simulink model "r2_1f_2x_4a_4k_r366"  (R2012b)
(part 4 of 95)

  xeng0/3(valid) -> vacc_tvg0/4(valid_in), snap_xeng0/2(we)
  [xeng_tvg_sel] -> xeng_tvg0/1(tvg_sel)
  [vacc_tvg_sel] -> vacc_tvg0/1(tvg_sel)
  Delay151/1(q) -> Delay83/1(d)
  Delay20/1(q) -> xeng_tvg0/2(sync)
  Delay21/1(q) -> xeng_tvg0/3(data_in)
  Delay22/1(q) -> xeng_tvg0/4(valid_in)
  Delay26/1(q) -> Delay151/1(d)
  gbe_rx_err_cnt0/1(sim_out) -> Terminator7/1
  Delay2/1(q) -> gbe_rx_err_cnt0/1(out_reg)
  Subsystem/2(rx_err_cnt) -> Delay2/1(d)
  Slice2/1 -> Delay117/1(d)
  Delay117/1(q) -> [loopback_mux_rst]
  Delay118/1(q) -> negedge_delay1/1(in)
  Slice8/1 -> Delay122/1(d)
  Delay122/1(q) -> [gbe_out_rst]
  16b_32b/1(Out1) -> snap_xeng0/1(din), vacc_tvg0/3(data_in)
  last_missing_ant0/1(sim_out) -> Terminator11/1
  Delay130/1(q) -> last_missing_ant0/1(out_reg)
  miss_cnt0/3(last_missed_ant) -> Convert2/1
  Slice14/1 -> Delay100/1(d)
  Delay100/1(q) -> [gbe_out_enable]
  spead_unpack0/8(hdr3_0x4102) -> pre_process0/7(hdr3)
  spead_unpack0/5(pkt_bad) -> Delay82/1(d), pre_process0/4(spead_err)
  Delay12/1(q) -> Subsystem4/8(overrun)
  [gbe_up0] -> Delay87/1(d)
  [gbe_rx0] -> Delay86/1(d)
  [gbe_rxvld0] -> delay46/1
  [gbe_rxdata0] -> delay45/1
  [gbe_rxeof0] -> delay47/1
  Delay87/1(q) -> Subsystem4/1(led_up)
  Delay86/1(q) -> Subsystem4/2(led_rx)
  delay45/1 -> spead_unpack0/1(pkt_data)
  delay46/1 -> spead_unpack0/2(pkt_valid)
  delay47/1 -> spead_unpack0/3(pkt_eof)
  vacc_tvg0/1(sync_out) -> vacc0/5(sync_in)
  vacc_tvg0/2(data_out) -> vacc0/6(data_in)
  vacc_tvg0/3(valid_out) -> vacc0/7(we)
  [acc_len] -> vacc0/4(acc_len)
  xeng0/4(mcnt_out) -> delay5/1
  vacc_cnt0/1(sim_out) -> Terminator10/1
  vacc_monitor/2(spec_cnt) -> vacc_cnt0/1(out_reg)
  vacc_err_cnt0/1(sim_out) -> Terminator1/1
  vacc_monitor/1(error_cnt) -> vacc_err_cnt0/1(out_reg)
  vacc0/1(new_acc) -> [new_acc0]
  [cnt_rst] -> vacc_monitor/1(cnt_rst)
  vacc0/7(timestamp) -> delay7/1
  [gbe_up0] -> Subsystem3/5(link_up)
  [gbe_tx0] -> Subsystem3/6(led_tx)
  [gbe_txd0] -> Subsystem3/1(data_in)
  [gbe_txvld0] -> Subsystem3/2(valid_in)
  [gbe_txip] -> Subsystem3/3(ip_in)
  [gbe_txeof0] -> Subsystem3/4(eof_in)
  [gbe_rxvld0] -> Delay25/1(d)
  [gbe_rxeof0] -> Delay18/1(d)
  Delay25/1(q) -> Subsystem/2(valid)
  Delay18/1(q) -> Subsystem/3(eof)
  [gbe_rx_bad0] -> Delay6/1(d)
  [gbe_rx_over0] -> Delay7/1(d)
  [gbe_rxip0] -> Delay53/1(d)
  [gbe_rxvld0] -> Delay59/1(d)
  [gbe_rxdata0] -> Delay70/1(d)
  [gbe_rxeof0] -> Delay29/1(d)
  Delay70/1(q) -> Subsystem4/3(data_in)
  Delay59/1(q) -> Subsystem4/4(valid_in)
  Delay53/1(q) -> Subsystem4/5(ip_in)
  Delay29/1(q) -> Subsystem4/6(eof_in)
  Constant1/1 -> Delay103/1(d)
  Delay80/1(q) -> Subsystem5/2(we)
  Delay81/1(q) -> Subsystem5/3(eof)
  Delay82/1(q) -> Subsystem5/4(flag)
  [gbe_tx_over0] -> gbe_err/4(overflow)
  [gbe_txeof0] -> gbe_err/3(eof)
  [gbe_txvld0] -> gbe_err/2(valid)
  Delay6/1(q) -> Subsystem/4(rx_bad_frame)
  Delay7/1(q) -> Subsystem/5(rx_overflow)
  [gbe_rx_bad0] -> Delay8/1(d)
  [gbe_rx_over0] -> Delay12/1(d)
  [gbe_tx_full0] -> Subsystem3/7(tx_full)
  [gbe_tx_over0] -> Subsystem3/8(tx_over)
  Delay56/1(q) -> xeng0/1(sync_in)
  Delay73/1(q) -> xeng0/2(ant)
  Delay74/1(q) -> xeng0/3(window_valid)
  Delay83/1(q) -> xeng0/4(mcnt_in)
  [gbe_out_rst] -> delay8/1
  [gbe_txd0] -> delay9/1
  [gbe_txvld0] -> delay10/1
  [gbe_txip] -> delay11/1
  [gbe_txport] -> delay12/1
  [gbe_txeof0] -> delay13/1
  gbe0/1 -> [gbe_up0]
  gbe0/2 -> [gbe_rx0]
  gbe0/3 -> [gbe_tx0]
  gbe0/4 -> [gbe_tx_full0]
  gbe0/5 -> [gbe_tx_over0]
  gbe0/12 -> [gbe_rx_over0]
  gbe0/11 -> [gbe_rx_bad0]
  gbe0/6 -> [gbe_rxdata0]
  gbe0/7 -> [gbe_rxvld0]
  gbe0/8 -> [gbe_rxip0]
  gbe0/9 -> [gbe_rxport0]
  gbe0/10 -> [gbe_rxeof0]
  [vacc_ld_arm] -> vacc0/2(arm)
  [vacc_ld_time] -> vacc0/3(load_time)
  [vacc_rst] -> vacc0/1(rst)
  vacc_ld_status0/1(sim_out) -> Terminator4/1
  delay5/1 -> vacc0/8(pcnt_in)
  vacc0/10(error_out) -> [vacc_err0]
  [new_acc0] -> vacc_monitor/2(new_acc)
  [vacc_err0] -> vacc_monitor/3(error)
  pkt_reord_devel2/2(data_out) -> snap_reord0/2(in_data), Delay21/1(d)
  Delay27/1(q) -> negedge_delay2/1(in)
  Delay96/1(q) -> negedge_delay3/1(in)
  Delay97/1(q) -> negedge_delay4/1(in)
  miss_cnt0/4(not_rcvd) -> [xeng_rx_err0]
  vacc0/2(data_out) -> delay4/1
  vacc0/4(valid_out) -> delay2/1
  vacc0/6(rb_done) -> delay6/1
  [vacc_ld_stat0] -> vacc_ld_status0/1(out_reg)
  vacc0/8(ld_status) -> [vacc_ld_stat0]
  [id0] -> pack_out0/6(xeng_id)
  [vacc_err0] -> snap_vacc0/4(stop)
  pack_out0/3(eof) -> Delay15/1(d)
  pack_out_err0/1(sim_out) -> Terminator6/1
  pack_out_cnt0/1(sim_out) -> Terminator5/1
  [cnt_rst] -> vacc_monitor2/1(cnt_rst)
  vacc_monitor2/1(pkt_cnt) -> pack_out_cnt0/1(out_reg)
  vacc_monitor2/2(error_cnt) -> pack_out_err0/1(out_reg)
  pack_out0/5(fetch) -> vacc0/9(re)
  delay4/1 -> snap_vacc0/1(din), pack_out0/1(data_in)
  delay2/1 -> snap_vacc0/2(we), pack_out0/2(valid_in)
  delay6/1 -> pack_out0/4(rb_done), snap_vacc0/3(trig)
  delay7/1 -> pack_out0/5(timestamp)
  pack_out0/1(data_out) -> Delay23/1(d)
  pack_out0/2(valid_out) -> Logical/2
  pack_out0/4(err) -> Delay34/1(d)
  Delay34/1(q) -> [pack_err0], vacc_monitor2/3(error)
  delay8/1 -> gbe0/1
  delay9/1 -> gbe0/2
  delay10/1 -> gbe0/3
  delay11/1 -> gbe0/4
  delay12/1 -> gbe0/5
  delay13/1 -> gbe0/6
  Constant2/1 -> gbe0/7
  Constant8/1 -> gbe0/8
  Delay46/1 -> pack_out0/3(pkt_rdy)
  Slice6/1 -> Delay44/1(d)
  Delay44/1(q) -> [flasher_en]
  negedge_delay3/1(out) -> front_panel/6(led2_red)
  negedge_delay4/1(out) -> front_panel/7(led3_red)
  [flasher_en] -> front_panel/1(flasher_en)
  [new_acc0] -> front_panel/2(sync)
  [x_sync0] -> front_panel/3(step)
  xstatus0/1(sim_out) -> Terminator24/1
  Subsystem6/1(status) -> xstatus0/1(out_reg)
  [clr_status] -> Subsystem6/1(clr)
  negedge_delay2/1(out) -> front_panel/4(led0_red)
  negedge_delay/1(out) -> front_panel/10(led6_green)
  negedge_delay1/1(out) -> front_panel/9(led5_green)
  Slice10/1 -> Delay13/1(d)
  Delay13/1(q) -> [clr_status]
  Inverter5/1 -> Subsystem6/2(gbe_down)
  [gbe_up0] -> Inverter5/1
  [vacc_err0] -> Subsystem6/10(vacc_err)
  [gbe_rx_bad0] -> Subsystem6/12(rx_bad_frame)
  [pack_err0] -> Subsystem6/15(pack_err)
  Subsystem3/1(data_out) -> snap_gbe_tx0/1(din)
  Subsystem3/2(we_out) -> snap_gbe_tx0/2(we)
  Subsystem3/3(trig_out) -> snap_gbe_tx0/3(trig)
  Subsystem4/1(data_out) -> snap_gbe_rx0/1(din)
  Subsystem4/2(we_out) -> snap_gbe_rx0/2(we)
  Subsystem4/3(trig_out) -> snap_gbe_rx0/3(trig)
  Delay16/1 -> [gbe_txvld0]
  Delay23/1(q) -> rate_ctrl0/1(din0)
  rate_ctrl0/2(valid) -> Delay16/1
  Constant22/1 -> [beng_data_id]
  rate_ctrl0/1(dout) -> Delay114/1
  Delay114/1 -> [gbe_txd0]
  err_clear_sim1/1 -> gbe_out_port/1(sim_1)
  gbe_out_port/1(in_reg) -> Delay9/1(d)
  Delay9/1(q) -> [gbe_out_txport]
  err_clear_sim5/1 -> gbe_out_ip/1(sim_1)
  gbe_out_ip/1(in_reg) -> Delay10/1(d)
  Delay10/1(q) -> [gbe_out_ip_addr]
  [gbe_out_txport] -> [gbe_txport]
  [gbe_out_ip_addr] -> [gbe_txip]
  [gbe_out_enable] -> Logical/1
  Constant24/1 -> [beng_time_id]
  Logical/1 -> rate_ctrl0/2(valid0)
  Delay15/1(q) -> vacc_monitor2/2(eof), rate_ctrl0/3(eof0)
  vacc0/5(pkt_rdy) -> rate_ctrl0/4(data_rdy0)
  spead_unpack0/1(pkt_start) -> Terminator28/1
  spead_unpack0/9(hdr4_0x4103) -> pre_process0/8(hdr4)
  pre_process0/9(dest_err) -> [rx_dest_err0]
  pre_process0/1(data_out) -> pkt_reord_devel2/1(din)
  pre_process0/2(valid) -> pkt_reord_devel2/2(valid_in)
  pre_process0/3(eof_out) -> pkt_reord_devel2/3(eof)
  pre_process0/4(timestamp) -> pkt_reord_devel2/4(time)
  pre_process0/5(feng_id) -> pkt_reord_devel2/5(ant)
  pre_process0/6(freq_out) -> pkt_reord_devel2/6(freq)
  pre_process0/8(spead_err_out) -> [spead_err0]
  pre_process0/7(adc_over) -> [adc_err0]
  pre_process0/10(fft_err) -> [fft_err0]
  pre_process0/11(feng_rx_err) -> [feng_rx_err0]
  pre_process0/12(nd_en) -> [noise_diode_en0]
  pkt_reord_devel2/7(err) -> Terminator2/1
  pre_process0/13(chksum_err) -> [feng_chk_err0]
  pre_process0/14(qdr_err) -> [feng_qdr_err0]
  [id0] -> pre_process0/9(board_id)
  err_clear_sim3/1 -> board_id/1(sim_1)
  Constant3/1 -> Delay72/1(d)
  Delay72/1(q) -> Subsystem1/1(In1)
  Subsystem1/1(Out1) -> [id0]
  Subsystem1/2(Out2) -> [id1]
  Subsystem1/3(Out3) -> [id2]
  Subsystem1/4(Out4) -> [id3]
  [id0] -> pkt_reord_devel2/8(board_id)
  pkt_reord_devel2/3(valid_out) -> snap_reord0/10(we), snap_reord0/3(in_valid), miss_cnt0/3(valid), Logical6/2, Delay22/1(d)
  pkt_reord_devel2/5(freq_out) -> Convert12/1
  Slice12/1 -> snap_reord0/7(in_feng_err)
  Slice16/1 -> snap_reord0/9(in_nd_on)
  Slice15/1 -> snap_reord0/8(in_adc_over)
  pkt_reord_devel2/6(flag_out) -> Slice11/1, Slice12/1, Slice15/1, Slice16/1
  Slice11/1 -> Logical6/1, snap_reord0/6(in_xeng_err), miss_cnt0/4(not rcvd)
  Logical6/1 -> snap_reord0/12(stop)
  miss_cnt1/2(missing_cnt) -> Convert4/1
  [cnt_rst] -> miss_cnt1/1(rst)
  miss_cnt1/1(spectr_cnt) -> Convert3/1
  pkt_reord_devel1/4(time_out) -> Slice21/1, Delay30/1(d)
  pkt_reord_devel1/1(sync_out) -> snap_reord1/11(trig), snap_reord1/1(in_sync), miss_cnt1/2(sync), Delay5/1(d)
  xeng_tvg1/1(sync_out) -> Delay32/1(d)
  xeng_tvg1/2(data_out) -> Delay36/1(d)
  xeng_tvg1/3(valid_out) -> Delay37/1(d)
  xeng1/1(sync_out) -> vacc_tvg1/2(sync_in)
  xeng1/2(acc) -> 16b_32b1/1(In1)
  xeng1/3(valid) -> vacc_tvg1/4(valid_in)
  [xeng_tvg_sel] -> xeng_tvg1/1(tvg_sel)
  [vacc_tvg_sel] -> vacc_tvg1/1(tvg_sel)
  Delay4/1(q) -> Delay38/1(d)
  Delay5/1(q) -> xeng_tvg1/2(sync)
  Delay11/1(q) -> xeng_tvg1/3(data_in)
  Delay14/1(q) -> xeng_tvg1/4(valid_in)
  Delay30/1(q) -> Delay4/1(d)
  16b_32b1/1(Out1) -> vacc_tvg1/3(data_in)
  miss_cnt1/3(last_missed_ant) -> Convert5/1
  vacc_tvg1/1(sync_out) -> vacc1/5(sync_in)
  vacc_tvg1/2(data_out) -> vacc1/6(data_in)
  vacc_tvg1/3(valid_out) -> vacc1/7(we)
  [acc_len] -> vacc1/4(acc_len)
  xeng1/4(mcnt_out) -> delay16/1
  vacc_monitor1/2(spec_cnt) -> vacc_cnt1/1(out_reg)
  vacc_monitor1/1(error_cnt) -> vacc_err_cnt1/1(out_reg)
  vacc1/1(new_acc) -> vacc_monitor1/2(new_acc), [new_acc1]
  [cnt_rst] -> vacc_monitor1/1(cnt_rst)
  vacc1/7(timestamp) -> delay18/1
  Delay32/1(q) -> xeng1/1(sync_in)
  Delay36/1(q) -> xeng1/2(ant)
  Delay37/1(q) -> xeng1/3(window_valid)
  Delay38/1(q) -> xeng1/4(mcnt_in)
  [vacc_ld_arm] -> vacc1/2(arm)
  [vacc_ld_time] -> vacc1/3(load_time)
  [vacc_rst] -> vacc1/1(rst)
  delay16/1 -> vacc1/8(pcnt_in)
  pkt_reord_devel1/2(data_out) -> snap_reord1/2(in_data), Delay11/1(d)
  miss_cnt1/4(not_rcvd) -> [xeng_rx_err1]
  vacc1/2(data_out) -> delay3/1
  vacc1/4(valid_out) -> delay1/1
  vacc1/6(rb_done) -> delay17/1
  vacc1/5(pkt_rdy) -> rate_ctrl1/4(data_rdy0)
  vacc1/8(ld_status) -> vacc_ld_status1/1(out_reg)
  [id1] -> pack_out1/6(xeng_id)
  vacc1/10(error_out) -> snap_vacc1/4(stop), vacc_monitor1/3(error), [vacc_err1]
  pack_out1/3(eof) -> Delay3/1(d)
  pack_out_err1/1(sim_out) -> Terminator31/1
  pack_out_cnt1/1(sim_out) -> Terminator29/1
  [cnt_rst] -> vacc_monitor3/1(cnt_rst)
  vacc_monitor3/1(pkt_cnt) -> pack_out_cnt1/1(out_reg)
  vacc_monitor3/2(error_cnt) -> pack_out_err1/1(out_reg)
  pack_out1/5(fetch) -> vacc1/9(re)
  delay3/1 -> pack_out1/1(data_in), snap_vacc1/1(din)
  delay1/1 -> pack_out1/2(valid_in), snap_vacc1/2(we)
  delay17/1 -> pack_out1/4(rb_done), snap_vacc1/3(trig)
  delay18/1 -> pack_out1/5(timestamp)
  pack_out1/1(data_out) -> Delay28/1(d)
  pack_out1/2(valid_out) -> Logical7/2
  Delay28/1(q) -> rate_ctrl1/1(din0)
  Logical7/1 -> rate_ctrl1/2(valid0)
  pack_out1/4(err) -> Delay31/1(d)
  Delay3/1(q) -> vacc_monitor3/2(eof), rate_ctrl1/3(eof0)
  Delay31/1(q) -> [pack_err1], vacc_monitor3/3(error)
  Delay42/1 -> pack_out1/3(pkt_rdy)
  [gbe_out_enable] -> Logical7/1
  pkt_reord_devel1/7(err) -> Terminator20/1
  [id1] -> pkt_reord_devel1/8(board_id)
  [flags1] -> pkt_reord_devel1/7(flag)
  pkt_reord_devel1/3(valid_out) -> snap_reord1/10(we), snap_reord1/3(in_valid), miss_cnt1/3(valid), Logical8/2, Delay14/1(d)
  pkt_reord_devel1/5(freq_out) -> Convert13/1
  Slice18/1 -> snap_reord1/7(in_feng_err)
  Slice20/1 -> snap_reord1/9(in_nd_on)
  Slice19/1 -> snap_reord1/8(in_adc_over)
  pkt_reord_devel1/6(flag_out) -> Slice20/1, Slice19/1, Slice18/1, Slice17/1
  Slice17/1 -> snap_reord1/6(in_xeng_err), miss_cnt1/4(not rcvd), Logical8/1
  Logical8/1 -> snap_reord1/12(stop)
  Constant12/1 -> vacc_time_msw/1(sim_1)
  Constant6/1 -> vacc_time_lsw/1(sim_1)
  vacc_time_msw/1(in_reg) -> Slice4/1, Slice13/1
  Slice13/1 -> Concat12/1
  vacc_time_lsw/1(in_reg) -> Concat12/2
  Slice4/1 -> [vacc_ld_arm]
  Concat12/1 -> [vacc_ld_time]
  rate_ctrl0/3(eof) -> Delay45/1
  rate_ctrl0/4(pkt_send0) -> Delay46/1
  Delay45/1 -> [gbe_txeof0]
  Delay40/1 -> [gbe_txvld1]
  rate_ctrl1/2(valid) -> Delay40/1
  rate_ctrl1/1(dout) -> Delay39/1
  Delay39/1 -> [gbe_txd1]
  rate_ctrl1/3(eof) -> Delay41/1
  rate_ctrl1/4(pkt_send0) -> Delay42/1
  Delay41/1 -> [gbe_txeof1]
  Subsystem8/1(rx_cnt) -> Delay68/1(d)
  [cnt_rst] -> Subsystem8/1(rst)
  spead_unpack1/3(valid64) -> Delay85/1(d), pre_process1/2(valid_in)
  spead_unpack1/6(hdr1_0x1600) -> pre_process1/5(hdr1)
  spead_unpack1/2(data64) -> pre_process1/1(data_in)
  spead_unpack1/4(eof64) -> Delay90/1(d), pre_process1/3(eof_in)
  spead_unpack1/7(hdr2_0x4101) -> pre_process1/6(hdr2)
  Subsystem8/2(err_cnt) -> Delay69/1(d)
  rx_cnt1/1(sim_out) -> Terminator32/1
  rx_err_cnt1/1(sim_out) -> Terminator33/1
  spead_unpack1/8(hdr3_0x4102) -> pre_process1/7(hdr3)
  spead_unpack1/5(pkt_bad) -> Delay91/1(d), pre_process1/4(spead_err)
  gbe1/6 -> Delay84/1(d)
  Delay84/1(q) -> spead_unpack1/1(pkt_data)
  Delay77/1(q) -> spead_unpack1/2(pkt_valid)
  Delay57/1(q) -> spead_unpack1/3(pkt_eof)
  Delay85/1(q) -> Subsystem8/2(we)
  Delay90/1(q) -> Subsystem8/3(eof)
  Delay91/1(q) -> Subsystem8/4(flag)
  spead_unpack1/1(pkt_start) -> Terminator34/1
  spead_unpack1/9(hdr4_0x4103) -> pre_process1/8(hdr4)
  pre_process1/9(dest_err) -> [rx_dest_err1]
  pre_process1/1(data_out) -> pkt_reord_devel1/1(din)
  pre_process1/2(valid) -> pkt_reord_devel1/2(valid_in)
  pre_process1/3(eof_out) -> pkt_reord_devel1/3(eof)
  pre_process1/4(timestamp) -> pkt_reord_devel1/4(time)
  pre_process1/5(feng_id) -> pkt_reord_devel1/5(ant)
  pre_process1/6(freq_out) -> pkt_reord_devel1/6(freq)
  pre_process1/8(spead_err_out) -> [spead_err1]
  pre_process1/7(adc_over) -> [adc_err1]
  pre_process1/10(fft_err) -> [fft_err1]
  pre_process1/11(feng_rx_err) -> [feng_rx_err1]
  pre_process1/12(nd_en) -> [noise_diode_en1]
  pre_process1/13(chksum_err) -> [feng_chk_err1]
  pre_process1/14(qdr_err) -> [feng_qdr_err1]
  [id1] -> pre_process1/9(board_id)
  [gbe_out_rst] -> delay21/1
  [gbe_txd1] -> delay22/1
  [gbe_txip] -> delay15/1
  [gbe_txport] -> delay19/1
  delay21/1 -> gbe1/1
  delay22/1 -> gbe1/2
  delay14/1 -> gbe1/3
  delay15/1 -> gbe1/4
  delay19/1 -> gbe1/5
  delay20/1 -> gbe1/6
  Constant9/1 -> gbe1/7
  Constant13/1 -> gbe1/8
  gbe_err1/1(tx_cnt) -> Delay98/1(d)
  Subsystem9/1(rx_cnt) -> Delay101/1(d)
  [cnt_rst] -> gbe_err1/1(rst)
  [cnt_rst] -> Subsystem9/1(rst)
  gbe_err1/2(err_cnt) -> Delay99/1(d)
  gbe_rx_cnt1/1(sim_out) -> Terminator37/1
  Delay98/1(q) -> gbe_tx_cnt1/1(out_reg)
  Delay99/1(q) -> gbe_tx_err_cnt1/1(out_reg)
  Delay101/1(q) -> gbe_rx_cnt1/1(out_reg)
  gbe_rx_err_cnt1/1(sim_out) -> Terminator38/1
  Delay93/1(q) -> gbe_rx_err_cnt1/1(out_reg)
  Subsystem9/2(rx_err_cnt) -> Delay93/1(d)
  gbe1/7 -> Delay94/1(d), Delay77/1(d)
  gbe1/10 -> Delay57/1(d), Delay92/1(d)
  Delay94/1(q) -> Subsystem9/2(valid)
  Delay92/1(q) -> Subsystem9/3(eof)
  gbe1/11 -> Delay95/1(d), [gbe_rx_bad1]
  gbe1/12 -> Delay102/1(d)
  gbe1/5 -> [gbe_tx_over1], gbe_err1/4(overflow)
  [gbe_txeof1] -> gbe_err1/3(eof), delay20/1
  [gbe_txvld1] -> gbe_err1/2(valid), delay14/1
  Delay95/1(q) -> Subsystem9/4(rx_bad_frame)
  Delay102/1(q) -> Subsystem9/5(rx_overflow)
  Delay103/1(q) -> Subsystem4/9(ack_in)
  miss_cnt2/2(missing_cnt) -> Convert7/1
  [cnt_rst] -> miss_cnt2/1(rst)
  miss_cnt2/1(spectr_cnt) -> Convert6/1
  pkt_reord_devel3/4(time_out) -> Slice27/1, Delay111/1(d)
  pkt_reord_devel3/1(sync_out) -> Delay133/1(d), snap_reord2/11(trig), snap_reord2/1(in_sync), miss_cnt2/2(sync)
  xeng_tvg2/1(sync_out) -> Delay113/1(d)
  xeng_tvg2/2(data_out) -> Delay119/1(d)
  xeng_tvg2/3(valid_out) -> Delay120/1(d)
  xeng2/1(sync_out) -> vacc_tvg2/2(sync_in)
  xeng2/2(acc) -> 16b_32b2/1(In1)
  xeng2/3(valid) -> vacc_tvg2/4(valid_in)
  [xeng_tvg_sel] -> xeng_tvg2/1(tvg_sel)
  [vacc_tvg_sel] -> vacc_tvg2/1(tvg_sel)
  Delay124/1(q) -> Delay121/1(d)
  Delay133/1(q) -> xeng_tvg2/2(sync)
  Delay107/1(q) -> xeng_tvg2/3(data_in)
  Delay108/1(q) -> xeng_tvg2/4(valid_in)
  Delay111/1(q) -> Delay124/1(d)
  16b_32b2/1(Out1) -> vacc_tvg2/3(data_in)
  miss_cnt2/3(last_missed_ant) -> Convert8/1
  vacc_tvg2/1(sync_out) -> vacc2/5(sync_in)
  vacc_tvg2/2(data_out) -> vacc2/6(data_in)
  vacc_tvg2/3(valid_out) -> vacc2/7(we)
  [acc_len] -> vacc2/4(acc_len)
  xeng2/4(mcnt_out) -> delay26/1
  vacc_cnt2/1(sim_out) -> Terminator55/1
  vacc_monitor4/2(spec_cnt) -> vacc_cnt2/1(out_reg)
  vacc_err_cnt2/1(sim_out) -> Terminator46/1
  vacc_monitor4/1(error_cnt) -> vacc_err_cnt2/1(out_reg)
  vacc2/1(new_acc) -> [new_acc2], vacc_monitor4/2(new_acc)
  [cnt_rst] -> vacc_monitor4/1(cnt_rst)
  vacc2/7(timestamp) -> delay28/1
  Delay113/1(q) -> xeng2/1(sync_in)
  Delay119/1(q) -> xeng2/2(ant)
  Delay120/1(q) -> xeng2/3(window_valid)
  Delay121/1(q) -> xeng2/4(mcnt_in)
  [vacc_ld_arm] -> vacc2/2(arm)
  [vacc_ld_time] -> vacc2/3(load_time)
  [vacc_rst] -> vacc2/1(rst)
  vacc_ld_status2/1(sim_out) -> Terminator43/1
  delay26/1 -> vacc2/8(pcnt_in)
  pkt_reord_devel3/2(data_out) -> snap_reord2/2(in_data), Delay107/1(d)
  miss_cnt2/4(not_rcvd) -> [xeng_rx_err2]
  vacc2/2(data_out) -> delay33/1
  vacc2/4(valid_out) -> delay23/1
  vacc2/6(rb_done) -> delay27/1
  vacc2/5(pkt_rdy) -> rate_ctrl2/4(data_rdy0)
  vacc2/8(ld_status) -> vacc_ld_status2/1(out_reg)
  [id2] -> pack_out2/6(xeng_id)
  vacc2/10(error_out) -> [vacc_err2], vacc_monitor4/3(error), snap_vacc2/4(stop)
  pack_out2/3(eof) -> Delay110/1(d)
  pack_out_err2/1(sim_out) -> Terminator47/1
  pack_out_cnt2/1(sim_out) -> Terminator45/1
  [cnt_rst] -> vacc_monitor5/1(cnt_rst)
  vacc_monitor5/1(pkt_cnt) -> pack_out_cnt2/1(out_reg)
  vacc_monitor5/2(error_cnt) -> pack_out_err2/1(out_reg)
  pack_out2/5(fetch) -> vacc2/9(re)
  delay33/1 -> snap_vacc2/1(din), pack_out2/1(data_in)
  delay23/1 -> snap_vacc2/2(we), pack_out2/2(valid_in)
  delay27/1 -> snap_vacc2/3(trig), pack_out2/4(rb_done)
  delay28/1 -> pack_out2/5(timestamp)
  pack_out2/1(data_out) -> Delay109/1(d)
  pack_out2/2(valid_out) -> Logical12/2
  Delay109/1(q) -> rate_ctrl2/1(din0)
  Logical12/1 -> rate_ctrl2/2(valid0)
  pack_out2/4(err) -> Delay112/1(d)
  Delay110/1(q) -> rate_ctrl2/3(eof0), vacc_monitor5/2(eof)
  Delay112/1(q) -> [pack_err2], vacc_monitor5/3(error)
  Delay127/1 -> pack_out2/3(pkt_rdy)
  [gbe_out_enable] -> Logical12/1
  pkt_reord_devel3/7(err) -> Terminator40/1
  [id2] -> pkt_reord_devel3/8(board_id)
  [flags2] -> pkt_reord_devel3/7(flag)
  pkt_reord_devel3/3(valid_out) -> Delay108/1(d), Logical13/2, snap_reord2/10(we), miss_cnt2/3(valid), snap_reord2/3(in_valid)
  pkt_reord_devel3/5(freq_out) -> Convert14/1
  Slice24/1 -> snap_reord2/7(in_feng_err)
  Slice26/1 -> snap_reord2/9(in_nd_on)
  Slice25/1 -> snap_reord2/8(in_adc_over)
  pkt_reord_devel3/6(flag_out) -> Slice26/1, Slice25/1, Slice23/1, Slice24/1
  Slice23/1 -> Logical13/1, snap_reord2/6(in_xeng_err), miss_cnt2/4(not rcvd)
  Logical13/1 -> snap_reord2/12(stop)
  Delay125/1 -> [gbe_txvld2]
  rate_ctrl2/2(valid) -> Delay125/1
  rate_ctrl2/1(dout) -> Delay123/1
  Delay123/1 -> [gbe_txd2]
  rate_ctrl2/3(eof) -> Delay126/1
  rate_ctrl2/4(pkt_send0) -> Delay127/1
  Delay126/1 -> [gbe_txeof2]
  Subsystem11/1(rx_cnt) -> Delay149/1(d)
  [cnt_rst] -> Subsystem11/1(rst)
  spead_unpack2/3(valid64) -> pre_process2/2(valid_in), Delay155/1(d)
  spead_unpack2/6(hdr1_0x1600) -> pre_process2/5(hdr1)
  spead_unpack2/2(data64) -> pre_process2/1(data_in)
  spead_unpack2/4(eof64) -> pre_process2/3(eof_in), Delay156/1(d)
  spead_unpack2/7(hdr2_0x4101) -> pre_process2/6(hdr2)
  Subsystem11/2(err_cnt) -> Delay150/1(d)
  rx_cnt2/1(sim_out) -> Terminator48/1
  rx_err_cnt2/1(sim_out) -> Terminator49/1
  Delay149/1(q) -> rx_cnt2/1(out_reg)
  Delay150/1(q) -> rx_err_cnt2/1(out_reg)
  spead_unpack2/8(hdr3_0x4102) -> pre_process2/7(hdr3)
  spead_unpack2/5(pkt_bad) -> pre_process2/4(spead_err), Delay157/1(d)
  gbe2/6 -> Delay154/1(d)
  Delay154/1(q) -> spead_unpack2/1(pkt_data)
  Delay153/1(q) -> spead_unpack2/2(pkt_valid)
  Delay139/1(q) -> spead_unpack2/3(pkt_eof)
  Delay155/1(q) -> Subsystem11/2(we)
  Delay156/1(q) -> Subsystem11/3(eof)
  Delay157/1(q) -> Subsystem11/4(flag)
  spead_unpack2/1(pkt_start) -> Terminator50/1
  spead_unpack2/9(hdr4_0x4103) -> pre_process2/8(hdr4)
  pre_process2/9(dest_err) -> [rx_dest_err2]
  pre_process2/1(data_out) -> pkt_reord_devel3/1(din)
  pre_process2/2(valid) -> pkt_reord_devel3/2(valid_in)
  pre_process2/3(eof_out) -> pkt_reord_devel3/3(eof)
  pre_process2/4(timestamp) -> pkt_reord_devel3/4(time)
  pre_process2/5(feng_id) -> pkt_reord_devel3/5(ant)
  pre_process2/6(freq_out) -> pkt_reord_devel3/6(freq)
  pre_process2/8(spead_err_out) -> [spead_err2]
  pre_process2/7(adc_over) -> [adc_err2]
  pre_process2/10(fft_err) -> [fft_err2]
  pre_process2/11(feng_rx_err) -> [feng_rx_err2]
  pre_process2/12(nd_en) -> [noise_diode_en2]
  pre_process2/13(chksum_err) -> [feng_chk_err2]
  pre_process2/14(qdr_err) -> [feng_qdr_err2]
  [id2] -> pre_process2/9(board_id)
  [gbe_out_rst] -> delay31/1
  [gbe_txd2] -> delay32/1
  [gbe_txip] -> delay25/1
  [gbe_txport] -> delay29/1
  delay31/1 -> gbe2/1
  delay32/1 -> gbe2/2
  delay24/1 -> gbe2/3
  delay25/1 -> gbe2/4
  delay29/1 -> gbe2/5
  delay30/1 -> gbe2/6
  Constant18/1 -> gbe2/7
  Constant14/1 -> gbe2/8
  gbe_err2/1(tx_cnt) -> Delay162/1(d)
  Subsystem12/1(rx_cnt) -> Delay105/1(d)
  [cnt_rst] -> gbe_err2/1(rst)
  [cnt_rst] -> Subsystem12/1(rst)
  gbe_err2/2(err_cnt) -> Delay163/1(d)
  gbe_tx_cnt2/1(sim_out) -> Terminator51/1
  gbe_tx_err_cnt2/1(sim_out) -> Terminator52/1
  gbe_rx_cnt2/1(sim_out) -> Terminator53/1
  Delay162/1(q) -> gbe_tx_cnt2/1(out_reg)
  Delay163/1(q) -> gbe_tx_err_cnt2/1(out_reg)
  Delay105/1(q) -> gbe_rx_cnt2/1(out_reg)
  gbe_rx_err_cnt2/1(sim_out) -> Terminator54/1
  Delay159/1(q) -> gbe_rx_err_cnt2/1(out_reg)
  Subsystem12/2(rx_err_cnt) -> Delay159/1(d)
  gbe2/7 -> Delay153/1(d), Delay160/1(d)
  gbe2/10 -> Delay158/1(d), Delay139/1(d)
  Delay160/1(q) -> Subsystem12/2(valid)
  Delay158/1(q) -> Subsystem12/3(eof)
  gbe2/11 -> [gbe_rx_bad2], Delay161/1(d)
  gbe2/12 -> Delay106/1(d)
  gbe2/5 -> [gbe_tx_over2], gbe_err2/4(overflow)
  [gbe_txeof2] -> delay30/1, gbe_err2/3(eof)
  [gbe_txvld2] -> delay24/1, gbe_err2/2(valid)
  Delay161/1(q) -> Subsystem12/4(rx_bad_frame)
  Delay106/1(q) -> Subsystem12/5(rx_overflow)
  miss_cnt3/2(missing_cnt) -> Convert10/1
  [cnt_rst] -> miss_cnt3/1(rst)
  miss_cnt3/1(spectr_cnt) -> Convert9/1
  pkt_reord_devel4/4(time_out) -> Slice36/1, Delay171/1(d)
  pkt_reord_devel4/1(sync_out) -> Delay188/1(d), snap_reord3/11(trig), snap_reord3/1(in_sync), miss_cnt3/2(sync)
  xeng_tvg3/1(sync_out) -> Delay173/1(d)
  xeng_tvg3/2(data_out) -> Delay176/1(d)
  xeng_tvg3/3(valid_out) -> Delay177/1(d)
  xeng3/1(sync_out) -> vacc_tvg3/2(sync_in)
  xeng3/2(acc) -> 16b_32b3/1(In1)
  xeng3/3(valid) -> vacc_tvg3/4(valid_in)
  [xeng_tvg_sel] -> xeng_tvg3/1(tvg_sel)
  [vacc_tvg_sel] -> vacc_tvg3/1(tvg_sel)
  Delay180/1(q) -> Delay178/1(d)
  Delay188/1(q) -> xeng_tvg3/2(sync)
  Delay167/1(q) -> xeng_tvg3/3(data_in)
  Delay168/1(q) -> xeng_tvg3/4(valid_in)
  Delay171/1(q) -> Delay180/1(d)
  16b_32b3/1(Out1) -> vacc_tvg3/3(data_in)
  miss_cnt3/3(last_missed_ant) -> Convert11/1
  vacc_tvg3/1(sync_out) -> vacc3/5(sync_in)
  vacc_tvg3/2(data_out) -> vacc3/6(data_in)
  vacc_tvg3/3(valid_out) -> vacc3/7(we)
  [acc_len] -> vacc3/4(acc_len)
  xeng3/4(mcnt_out) -> delay37/1
  vacc_monitor6/2(spec_cnt) -> vacc_cnt3/1(out_reg)
  vacc_monitor6/1(error_cnt) -> vacc_err_cnt3/1(out_reg)
  vacc3/1(new_acc) -> vacc_monitor6/2(new_acc), [new_acc3]
  [cnt_rst] -> vacc_monitor6/1(cnt_rst)
  vacc3/7(timestamp) -> delay39/1
  Delay173/1(q) -> xeng3/1(sync_in)
  Delay176/1(q) -> xeng3/2(ant)
  Delay177/1(q) -> xeng3/3(window_valid)
  Delay178/1(q) -> xeng3/4(mcnt_in)
  [vacc_ld_arm] -> vacc3/2(arm)
  [vacc_ld_time] -> vacc3/3(load_time)
  [vacc_rst] -> vacc3/1(rst)
  delay37/1 -> vacc3/8(pcnt_in)
  pkt_reord_devel4/2(data_out) -> snap_reord3/2(in_data), Delay167/1(d)
  miss_cnt3/4(not_rcvd) -> [xeng_rx_err3]
  vacc3/2(data_out) -> delay44/1
  vacc3/4(valid_out) -> delay34/1
  vacc3/6(rb_done) -> delay38/1
  vacc3/5(pkt_rdy) -> rate_ctrl3/4(data_rdy0)
  vacc3/8(ld_status) -> vacc_ld_status3/1(out_reg)
  [id3] -> pack_out3/6(xeng_id)
  vacc3/10(error_out) -> snap_vacc3/4(stop), vacc_monitor6/3(error), [vacc_err3]
  pack_out3/3(eof) -> Delay170/1(d)
  pack_out_err3/1(sim_out) -> Terminator64/1
  pack_out_cnt3/1(sim_out) -> Terminator62/1
  [cnt_rst] -> vacc_monitor7/1(cnt_rst)
  vacc_monitor7/1(pkt_cnt) -> pack_out_cnt3/1(out_reg)
  vacc_monitor7/2(error_cnt) -> pack_out_err3/1(out_reg)
  pack_out3/5(fetch) -> vacc3/9(re)
  delay44/1 -> pack_out3/1(data_in), snap_vacc3/1(din)
  delay34/1 -> pack_out3/2(valid_in), snap_vacc3/2(we)
  delay38/1 -> pack_out3/4(rb_done), snap_vacc3/3(trig)
  delay39/1 -> pack_out3/5(timestamp)
  pack_out3/1(data_out) -> Delay169/1(d)
  pack_out3/2(valid_out) -> Logical16/2
  Delay169/1(q) -> rate_ctrl3/1(din0)
  Logical16/1 -> rate_ctrl3/2(valid0)
  pack_out3/4(err) -> Delay172/1(d)
  Delay170/1(q) -> vacc_monitor7/2(eof), rate_ctrl3/3(eof0)
  Delay172/1(q) -> [pack_err3], vacc_monitor7/3(error)
  Delay183/1 -> pack_out3/3(pkt_rdy)
  [gbe_out_enable] -> Logical16/1
  pkt_reord_devel4/7(err) -> Terminator57/1
  [id3] -> pkt_reord_devel4/8(board_id)
  [flags3] -> pkt_reord_devel4/7(flag)
  pkt_reord_devel4/3(valid_out) -> snap_reord3/10(we), snap_reord3/3(in_valid), miss_cnt3/3(valid), Logical17/2, Delay168/1(d)
  pkt_reord_devel4/5(freq_out) -> Convert15/1
  Slice33/1 -> snap_reord3/7(in_feng_err)
  Slice35/1 -> snap_reord3/9(in_nd_on)
  Slice34/1 -> snap_reord3/8(in_adc_over)
  pkt_reord_devel4/6(flag_out) -> Slice35/1, Slice34/1, Slice33/1, Slice32/1
  Slice32/1 -> snap_reord3/6(in_xeng_err), miss_cnt3/4(not rcvd), Logical17/1
  Logical17/1 -> snap_reord3/12(stop)
  Delay181/1 -> [gbe_txvld3]
  rate_ctrl3/2(valid) -> Delay181/1
  rate_ctrl3/1(dout) -> Delay179/1
  Delay179/1 -> [gbe_txd3]
  rate_ctrl3/3(eof) -> Delay182/1
  rate_ctrl3/4(pkt_send0) -> Delay183/1
  Delay182/1 -> [gbe_txeof3]
  Subsystem14/1(rx_cnt) -> Delay195/1(d)
  [cnt_rst] -> Subsystem14/1(rst)
  spead_unpack3/3(valid64) -> pre_process3/2(valid_in), Delay200/1(d)
  spead_unpack3/6(hdr1_0x1600) -> pre_process3/5(hdr1)
  spead_unpack3/2(data64) -> pre_process3/1(data_in)
  spead_unpack3/4(eof64) -> pre_process3/3(eof_in), Delay201/1(d)
  spead_unpack3/7(hdr2_0x4101) -> pre_process3/6(hdr2)
  Subsystem14/2(err_cnt) -> Delay196/1(d)
  Delay195/1(q) -> rx_cnt3/1(out_reg)
  Delay196/1(q) -> rx_err_cnt3/1(out_reg)
  spead_unpack3/8(hdr3_0x4102) -> pre_process3/7(hdr3)
  spead_unpack3/5(pkt_bad) -> pre_process3/4(spead_err), Delay202/1(d)
  gbe3/6 -> Delay199/1(d)
  Delay199/1(q) -> spead_unpack3/1(pkt_data)
  Delay198/1(q) -> spead_unpack3/2(pkt_valid)
  Delay194/1(q) -> spead_unpack3/3(pkt_eof)
  Delay200/1(q) -> Subsystem14/2(we)
  Delay201/1(q) -> Subsystem14/3(eof)
  Delay202/1(q) -> Subsystem14/4(flag)
  spead_unpack3/1(pkt_start) -> Terminator67/1
  spead_unpack3/9(hdr4_0x4103) -> pre_process3/8(hdr4)
  pre_process3/9(dest_err) -> [rx_dest_err3], snap_unpack3/9(in_dest_err), Logical1/2
  pre_process3/1(data_out) -> snap_unpack3/1(in_data), pkt_reord_devel4/1(din)
  pre_process3/2(valid) -> snap_unpack3/2(in_valid), snap_unpack3/15(we), pkt_reord_devel4/2(valid_in)
  pre_process3/3(eof_out) -> pkt_reord_devel4/3(eof), snap_unpack3/16(trig), snap_unpack3/3(in_eof)
  pre_process3/4(timestamp) -> pkt_reord_devel4/4(time), Slice29/1
  pre_process3/5(feng_id) -> pkt_reord_devel4/5(ant), Slice30/1
  pre_process3/6(freq_out) -> pkt_reord_devel4/6(freq), Slice31/1
  pre_process3/8(spead_err_out) -> snap_unpack3/8(in_spead_err), Logical1/1, [spead_err3]
  pre_process3/7(adc_over) -> snap_unpack3/7(in_adc_over), [adc_err3]
  pre_process3/11(feng_rx_err) -> snap_unpack3/11(in_feng_rx_err), [feng_rx_err3]
  pre_process3/12(nd_en) -> snap_unpack3/12(in_nd_en), [noise_diode_en3]
  pre_process3/13(chksum_err) -> snap_unpack3/13(in_chksum_err), [feng_chk_err3]
  pre_process3/14(qdr_err) -> [feng_qdr_err3], snap_unpack3/14(in_feng_qdr_err)
  [id3] -> pre_process3/9(board_id)
  [gbe_out_rst] -> delay42/1
  [gbe_txd3] -> delay43/1
  [gbe_txip] -> delay36/1
  [gbe_txport] -> delay40/1
  delay42/1 -> gbe3/1
  delay43/1 -> gbe3/2
  delay35/1 -> gbe3/3
  delay36/1 -> gbe3/4
  delay40/1 -> gbe3/5
  delay41/1 -> gbe3/6
  Constant23/1 -> gbe3/7
  Constant19/1 -> gbe3/8
  gbe_err3/1(tx_cnt) -> Delay207/1(d)
  Subsystem15/1(rx_cnt) -> Delay165/1(d)
  [cnt_rst] -> gbe_err3/1(rst)
  [cnt_rst] -> Subsystem15/1(rst)
  gbe_err3/2(err_cnt) -> Delay208/1(d)
  gbe_tx_cnt3/1(sim_out) -> Terminator68/1
  gbe_tx_err_cnt3/1(sim_out) -> Terminator69/1
  gbe_rx_cnt3/1(sim_out) -> Terminator70/1
  Delay207/1(q) -> gbe_tx_cnt3/1(out_reg)
  Delay208/1(q) -> gbe_tx_err_cnt3/1(out_reg)
  Delay165/1(q) -> gbe_rx_cnt3/1(out_reg)
  gbe_rx_err_cnt3/1(sim_out) -> Terminator71/1
  Delay204/1(q) -> gbe_rx_err_cnt3/1(out_reg)
  Subsystem15/2(rx_err_cnt) -> Delay204/1(d)
  gbe3/7 -> Delay205/1(d), Delay198/1(d)
  gbe3/10 -> Delay194/1(d), Delay203/1(d)
  Delay205/1(q) -> Subsystem15/2(valid)
  Delay203/1(q) -> Subsystem15/3(eof)
  gbe3/11 -> [gbe_rx_bad3], Delay206/1(d)
  gbe3/12 -> Delay166/1(d)
  gbe3/5 -> [gbe_tx_over3], gbe_err3/4(overflow)
  [gbe_txeof3] -> gbe_err3/3(eof), delay41/1
  [gbe_txvld3] -> gbe_err3/2(valid), delay35/1
  Delay206/1(q) -> Subsystem15/4(rx_bad_frame)
  Delay166/1(q) -> Subsystem15/5(rx_overflow)
  gbe1/1 -> [gbe_up1]
  gbe2/1 -> [gbe_up2]
  gbe3/1 -> [gbe_up3]
  [spead_err0] -> Subsystem6/11(rx_bad_pkt)
  [xeng_rx_err0] -> Subsystem6/14(xeng_bad_dat)
  [gbe_tx_over0] -> Subsystem6/13(tx_over)
  [rx_dest_err0] -> Subsystem6/3(rx_dest_err)
  [feng_rx_err0] -> Subsystem6/4(feng_rx_err)
  [fft_err0] -> Subsystem6/5(fft_err)
  [feng_qdr_err0] -> Subsystem6/6(feng_qdr_err)
  [feng_chk_err0] -> Subsystem6/7(feng_chk_err)
  [adc_err0] -> Subsystem6/8(adc_over)
  [noise_diode_en0] -> Subsystem6/9(noise_diode_en)
  Subsystem6/4(flags) -> [flags0]
  Subsystem6/2(data_in_bad) -> [dat_in_bad0]
  Subsystem6/3(err) -> [err0]
  xstatus1/1(sim_out) -> Terminator27/1
  Subsystem7/1(status) -> xstatus1/1(out_reg)
  [clr_status] -> Subsystem7/1(clr)
  Inverter6/1 -> Subsystem7/2(gbe_down)
  [gbe_up1] -> Inverter6/1
  [vacc_err1] -> Subsystem7/10(vacc_err)
  [gbe_rx_bad1] -> Subsystem7/12(rx_bad_frame)
  [pack_err1] -> Subsystem7/15(pack_err)
  [spead_err1] -> Subsystem7/11(rx_bad_pkt)
  [xeng_rx_err1] -> Subsystem7/14(xeng_bad_dat)
  [gbe_tx_over1] -> Subsystem7/13(tx_over)
  [rx_dest_err1] -> Subsystem7/3(rx_dest_err)
  [feng_rx_err1] -> Subsystem7/4(feng_rx_err)
  [fft_err1] -> Subsystem7/5(fft_err)
  [feng_qdr_err1] -> Subsystem7/6(feng_qdr_err)
  [feng_chk_err1] -> Subsystem7/7(feng_chk_err)
  [adc_err1] -> Subsystem7/8(adc_over)
  [noise_diode_en1] -> Subsystem7/9(noise_diode_en)
  Subsystem7/4(flags) -> [flags1]
  Subsystem7/2(data_in_bad) -> [dat_in_bad1]
  Subsystem7/3(err) -> [err1]
  [clr_status] -> Subsystem10/1(clr)
  Inverter1/1 -> Subsystem10/2(gbe_down)
  [gbe_up2] -> Inverter1/1
  [vacc_err2] -> Subsystem10/10(vacc_err)
  [gbe_rx_bad2] -> Subsystem10/12(rx_bad_frame)
  [pack_err2] -> Subsystem10/15(pack_err)
  [spead_err2] -> Subsystem10/11(rx_bad_pkt)
  [xeng_rx_err2] -> Subsystem10/14(xeng_bad_dat)
  [gbe_tx_over2] -> Subsystem10/13(tx_over)
  [rx_dest_err2] -> Subsystem10/3(rx_dest_err)
  [feng_rx_err2] -> Subsystem10/4(feng_rx_err)
  [fft_err2] -> Subsystem10/5(fft_err)
  [feng_qdr_err2] -> Subsystem10/6(feng_qdr_err)
  [feng_chk_err2] -> Subsystem10/7(feng_chk_err)
  [adc_err2] -> Subsystem10/8(adc_over)
  [noise_diode_en2] -> Subsystem10/9(noise_diode_en)
  Subsystem10/4(flags) -> [flags2]
  Subsystem10/2(data_in_bad) -> [dat_in_bad2]
  Subsystem10/3(err) -> [err2]
  xstatus3/1(sim_out) -> Terminator18/1
  [clr_status] -> Subsystem13/1(clr)
  Inverter2/1 -> Subsystem13/2(gbe_down)
  [gbe_up1] -> Inverter2/1
  [vacc_err1] -> Subsystem13/10(vacc_err)
  [gbe_rx_bad1] -> Subsystem13/12(rx_bad_frame)
  [pack_err1] -> Subsystem13/15(pack_err)
  [spead_err1] -> Subsystem13/11(rx_bad_pkt)
  [xeng_rx_err1] -> Subsystem13/14(xeng_bad_dat)
  [gbe_tx_over1] -> Subsystem13/13(tx_over)
  [rx_dest_err1] -> Subsystem13/3(rx_dest_err)
  [feng_rx_err1] -> Subsystem13/4(feng_rx_err)
  [fft_err1] -> Subsystem13/5(fft_err)
  [feng_qdr_err1] -> Subsystem13/6(feng_qdr_err)
  [feng_chk_err1] -> Subsystem13/7(feng_chk_err)
  [adc_err1] -> Subsystem13/8(adc_over)
  [noise_diode_en1] -> Subsystem13/9(noise_diode_en)
  Subsystem13/4(flags) -> [flags3]
  Subsystem13/2(data_in_bad) -> [dat_in_bad3]
  Subsystem13/3(err) -> [err3]
  [flags0] -> pkt_reord_devel2/7(flag)
  Delay209/1(q) -> negedge_delay5/1(in)
  Delay210/1(q) -> negedge_delay6/1(in)
  negedge_delay6/1(out) -> front_panel/8(led4_green)
  negedge_delay5/1(out) -> front_panel/5(led1_red)
  Delay211/1(q) -> negedge_delay7/1(in)
  negedge_delay7/1(out) -> front_panel/11(led7_green)
  [err0] -> Delay27/1(d)
  [dat_in_bad0] -> Inverter3/1
  [dat_in_bad1] -> Inverter4/1
  [dat_in_bad2] -> Inverter7/1
  [dat_in_bad3] -> Inverter8/1
  Inverter3/1 -> Delay210/1(d)
  Inverter4/1 -> Delay118/1(d)
  Inverter7/1 -> Delay17/1(d)
  Inverter8/1 -> Delay211/1(d)
  [err1] -> Delay209/1(d)
  [err2] -> Delay96/1(d)
  [err3] -> Delay97/1(d)
  pre_process3/10(fft_err) -> snap_unpack3/10(in_fft_err), [fft_err3]
  Logical1/1 -> snap_unpack3/17(stop)
  Slice29/1 -> snap_unpack3/4(in_time)
  Slice30/1 -> snap_unpack3/5(in_feng_id)
  Slice31/1 -> snap_unpack3/6(in_freq)
  rx_cnt3/1(sim_out) -> Terminator65/1
  rx_err_cnt3/1(sim_out) -> Terminator66/1
  gbe_tx_cnt1/1(sim_out) -> Terminator35/1
  gbe_tx_err_cnt1/1(sim_out) -> Terminator36/1
  Delay68/1(q) -> rx_cnt1/1(out_reg)
  Delay69/1(q) -> rx_err_cnt1/1(out_reg)
  vacc_cnt1/1(sim_out) -> Terminator8/1
  vacc_ld_status1/1(sim_out) -> Terminator23/1
  vacc_err_cnt1/1(sim_out) -> Terminator3/1
  vacc_err_cnt3/1(sim_out) -> Terminator63/1
  vacc_cnt3/1(sim_out) -> Terminator72/1
  vacc_ld_status3/1(sim_out) -> Terminator60/1
  Subsystem13/1(status) -> xstatus3/1(out_reg)
  Subsystem10/1(status) -> xstatus2/1(out_reg)
  xstatus2/1(sim_out) -> Terminator9/1
  Slice21/1 -> snap_reord1/4(in_time)
  Convert13/1 -> snap_reord1/5(in_freq)
  Slice27/1 -> snap_reord2/4(in_time)
  Convert14/1 -> snap_reord2/5(in_freq)
  Slice36/1 -> snap_reord3/4(in_time)
  Convert15/1 -> snap_reord3/5(in_freq)
  Slice38/1 -> snap_reord0/4(in_time)
  Convert12/1 -> snap_reord0/5(in_freq)
  Convert/1 -> Delay61/1(d)
  Convert1/1 -> Delay62/1(d)
  Convert2/1 -> Delay130/1(d)
  pkt_reord_cnt1/1(sim_out) -> Terminator19/1
  pkt_reord_err1/1(sim_out) -> Terminator21/1
  Delay24/1(q) -> pkt_reord_cnt1/1(out_reg)
  Delay33/1(q) -> pkt_reord_err1/1(out_reg)
  last_missing_ant1/1(sim_out) -> Terminator12/1
  Delay1/1(q) -> last_missing_ant1/1(out_reg)
  Convert3/1 -> Delay24/1(d)
  Convert4/1 -> Delay33/1(d)
  Convert5/1 -> Delay1/1(d)
  pkt_reord_cnt2/1(sim_out) -> Terminator30/1
  pkt_reord_err2/1(sim_out) -> Terminator39/1
  Delay43/1(q) -> pkt_reord_cnt2/1(out_reg)
  Delay47/1(q) -> pkt_reord_err2/1(out_reg)
  last_missing_ant2/1(sim_out) -> Terminator22/1
  Delay35/1(q) -> last_missing_ant2/1(out_reg)
  Convert6/1 -> Delay43/1(d)
  Convert7/1 -> Delay47/1(d)
  Convert8/1 -> Delay35/1(d)
  pkt_reord_cnt3/1(sim_out) -> Terminator42/1
  pkt_reord_err3/1(sim_out) -> Terminator44/1
  Delay49/1(q) -> pkt_reord_cnt3/1(out_reg)
  Delay50/1(q) -> pkt_reord_err3/1(out_reg)
  last_missing_ant3/1(sim_out) -> Terminator41/1
  Delay48/1(q) -> last_missing_ant3/1(out_reg)
  Convert9/1 -> Delay49/1(d)
  Convert10/1 -> Delay50/1(d)
  Convert11/1 -> Delay48/1(d)
